simulink model "untitled1"  (R2018b)
settings: Solver=VariableStepAuto  StartTime=0.0  StopTime=0  RelTol=1e-3
libraries: commrandsrc3 x1
settings Model: Creator=DSP_26  LastModifiedBy=DSP_26

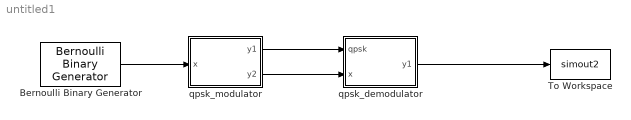
== system untitled1 ==
  Bernoulli Binary Generator : commrandsrc3/Bernoulli Binary Generator  ProbabilityOfZero=0.5  SeedSource=Auto  Seed=0  SampleTime=1  SamplesPerFrame=10000  OutputDataType=double  SimulateUsing=Interpreted execution
  To Workspace : ToWorkspace  VariableName=simout2  SampleTime=-1
      settings: Save2DSignal=2-D array (concatenate along first dimension)
  qpsk_demodulator : MATLAB Function  TreatAsAtomicUnit=on
  qpsk_modulator : MATLAB Function  TreatAsAtomicUnit=on
  wires:
  Bernoulli Binary Generator/1 -> qpsk_modulator/1(x)
  qpsk_demodulator/1(y1) -> To Workspace/1
  qpsk_modulator/1(y1) -> qpsk_demodulator/1(qpsk)
  qpsk_modulator/2(y2) -> qpsk_demodulator/2(x)

== matlab function untitled1/qpsk_demodulator ==
  data: qpsk input; y1 output; x input
function y1 = qpsk_demodulator(qpsk,x)
perror = zeros(1,7);
snrd = zeros(1,7);
a=0;
for r=2:7
    a = a + 4;
    snrd(r) = a;
end
snrl = zeros(1,7);
for r=1:7
    cnoise = randn(1,5000) + 1j*randn(1,5000);
    h = randn(1,5000) + 1j*randn(1,5000);
    snrl(r) = 10^(snrd(r)/10);
    sigma = sqrt(10.^(-snrl(r)/10));
    y = h.*qpsk + sigma*cnoise;
    y = y./h;
    qpsk1 = zeros(1,10000);
    k=1;
    for n=1:1:5000
        if(real(y(n))>0 && imag(y(n))>0)
            qpsk1(k) = 0;
            qpsk1(k+1) = 0;
        elseif(real(y(n))<0 && imag(y(n))>0)
            qpsk1(k) = 0;
            qpsk1(k+1) = 1;
        elseif(real(y(n))<0 && imag(y(n))<0)
            qpsk1(k) = 1;
            qpsk1(k+1) = 0;
        else
            qpsk1(k) = 1;
            qpsk1(k+1) = 1;
        end
        k=k+2;
    end
    perror(r) = mean(abs(x-qpsk1));  
end
y1 = perror;

== matlab function untitled1/qpsk_modulator ==
  data: x input; y1 output; y2 output
function [y1,y2] = qpsk_modulator(x)
x = transpose(x);
qpsk = zeros(1,5000) + 1j*zeros(1,5000);
k=1;
for i=1:2:10000
    if x(i)==0 && x(i+1)==0
        qpsk(k)=1+1j;
    elseif x(i)==0 && x(i+1)==1
        qpsk(k)=-1+1j;
    elseif x(i)==1 && x(i+1)==0
        qpsk(k)=-1-1j;
    else
        qpsk(k)=1-1j;
    end
    k=k+1;
end
y1 = qpsk;
y2 = x;
